simulink model "MVDR_example_hdl_4x4_partial_systolic"  (R2020b)
settings: Solver=FixedStepDiscrete  StartTime=0.0  StopTime=stoptime  RelTol=1e-3
InitFcn:
  | model_init
values from neighbouring files (symbols this model uses):
  movavg_bitshift = nextpow2(sqrt(windowSize))    [model_init.m]
  mvdrPipelineDelay = covMatDelay+movAvgDelay+matrixDivDelay+normResponseDelay    [model_init.m]
  numArrayElements = 4    [model_init.m]
  srcAngles = [20 60]    [model_init.m]
  sv = step(steeringVector,fc,[scanAngle; 0])    [model_init.m]
  Ts = 1/fs    (= 7.8125e-09)    [model_init.m]
  windowSize = 1024    [model_init.m]
libraries: hdlsllib x11, simulink x4, commfilt2 x4, commrfcorlib x3, commsync2 x3, commrflib2 x2, commrandsrc3 x2, phasedtxrxlib x2, commdigbbndcpm2 x1, embsystolicmatrixops x1, embreciprocals x1, commdigbbndpm3 x1
Description:
  | MVDR HDL 4x4 systolic testbench
settings Model: DataTypeOverride=Off  Creator=The MathWorks, Inc.  LastModifiedBy=tmealey
settings DataIOCC: LimitDataPoints=on  SaveFormat=Array  SaveOutput=off  SaveTime=off  ReturnWorkspaceOutputs=off
settings OptimizationCC: BlockReduction=off  ConditionallyExecuteInputs=off  DefaultParameterBehavior=Inlined  LifeSpan=inf
settings DebuggingCC: ReadBeforeWriteMsg=DisableAll  WriteAfterWriteMsg=DisableAll  WriteAfterReadMsg=DisableAll  AlgebraicLoopMsg=error  UnderspecifiedInitializationDetection=Classic  MergeDetectMultiDrivingBlocksExec=none  SolverPrmCheckMsg=warning  SingleTaskRateTransMsg=error  ParameterPrecisionLossMsg=none  AllowSymbolicDim=off  SFUnexpectedBacktrackingDiag=warning  SFNoUnconditionalDefaultTransitionDiag=warning  SFExecutionAtInitializationDiag=none  ArithmeticOperatorsInVariantConditions=warning
settings HardwareCC: ProdBitPerPointer=32  ProdBitPerSizeT=32  ProdBitPerPtrDiffT=32  ProdLargestAtomicFloat=None  ProdIntDivRoundTo=Undefined  ProdEndianess=Unspecified  ProdWordSize=32  ProdHWDeviceType=ASIC/FPGA->ASIC/FPGA  TargetBitPerPointer=64  TargetBitPerSizeT=64  TargetBitPerPtrDiffT=64  TargetLongLongMode=on  TargetIntDivRoundTo=Zero  TargetEndianess=LittleEndian  TargetWordSize=64  TargetHWDeviceType=Custom Processor->MATLAB Host Computer  ProdEqTarget=off
settings ModelReferenceCC: PropagateSignalLabelsOutOfModel=off
settings SFSimCC: SimUseLocalCustomCode=off  CustomCodeUndefinedFunction=UseInterfaceOnly
settings RTWCC: RTWUseLocalCustomCode=off
settings CodeAppCC: StateflowObjectComments=on
settings GRTTargetCC: TargetLangStandard=C89/C90 (ANSI)
settings ConfigComp: CovMetricSettings=dw  CovSaveCumulativeToWorkspaceVar=on  CovSaveSingleToWorkspaceVar=on  CovExternalEMLEnable=off  CovSFcnEnable=off

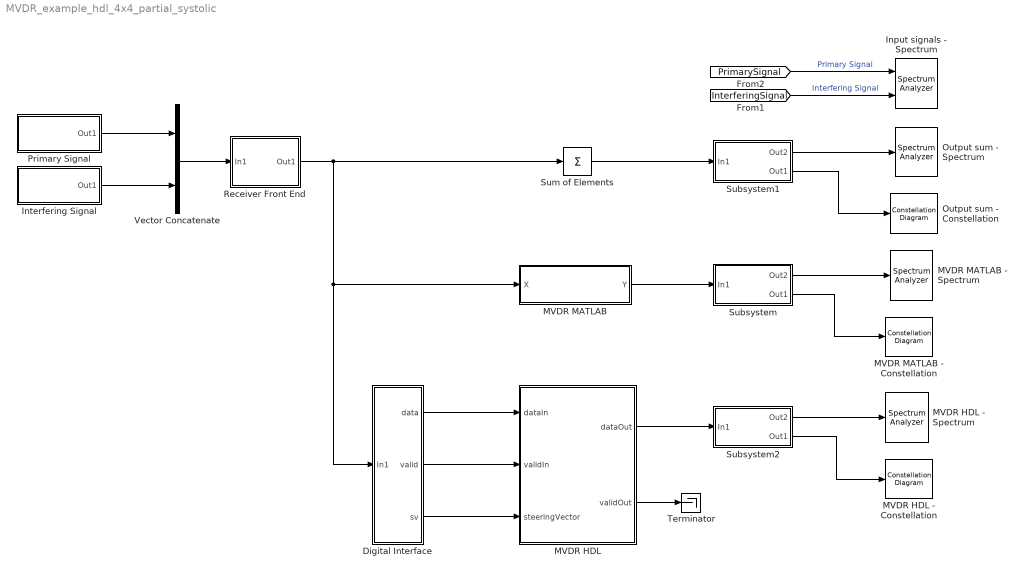
== system MVDR_example_hdl_4x4_partial_systolic ==
  Digital Interface : Subsystem
  Input signals - Spectrum : SpectrumAnalyzer  NumInputPorts=2
  Interfering Signal : Subsystem
      mask Display: disp('Interfering\nSignal')
  MVDR HDL : Subsystem
  MVDR HDL - Constellation : ConstellationDiagram
  MVDR HDL - Spectrum : SpectrumAnalyzer
  MVDR MATLAB : Subsystem
  MVDR MATLAB - Constellation : ConstellationDiagram
  MVDR MATLAB - Spectrum : SpectrumAnalyzer
  Output sum - Constellation : ConstellationDiagram
  Output sum - Spectrum : SpectrumAnalyzer
  Primary Signal : Subsystem
      mask Display: disp('Primary\nSignal')
  Receiver Front End : Subsystem
  Subsystem : Subsystem
  Subsystem1 : Subsystem
  Subsystem2 : Subsystem
  Sum of Elements : Sum  Inputs=+  CollapseMode=Specified dimension  CollapseDim=2
  Terminator : Terminator
  Vector Concatenate : Concatenate  Mode=Multidimensional array  ConcatenateDimension=2
  wires:
  MVDR HDL/2(validOut) -> Terminator/1
  MVDR MATLAB/1(Y) -> Subsystem/1(In1)
  Interfering Signal/1(Out1) -> Vector Concatenate/2
  Primary Signal/1(Out1) -> Vector Concatenate/1
  [InterferingSignal] -> Input signals - Spectrum/2  "Interfering Signal"
  Subsystem/2(Out1) -> MVDR MATLAB - Constellation/1
  Subsystem/1(Out2) -> MVDR MATLAB - Spectrum/1
  Sum of Elements/1 -> Subsystem1/1(In1)
  Subsystem1/1(Out2) -> Output sum - Spectrum/1
  Subsystem1/2(Out1) -> Output sum - Constellation/1
  MVDR HDL/1(dataOut) -> Subsystem2/1(In1)
  Subsystem2/1(Out2) -> MVDR HDL - Spectrum/1
  Subsystem2/2(Out1) -> MVDR HDL - Constellation/1
  [PrimarySignal] -> Input signals - Spectrum/1  "Primary Signal"
  Digital Interface/1(data) -> MVDR HDL/1(dataIn)
  Digital Interface/2(valid) -> MVDR HDL/2(validIn)
  Digital Interface/3(sv) -> MVDR HDL/3(steeringVector)
  Receiver Front End/1(Out1) -> MVDR MATLAB/1(X), Digital Interface/1(In1), Sum of Elements/1
  Vector Concatenate/1 -> Receiver Front End/1(In1)

== system MVDR_example_hdl_4x4_partial_systolic/Digital Interface ==
  In1 : Inport
  Constant1 : Constant  Value=true  SampleTime=-1
  Constant2 : Constant  Value=sv  SampleTime=-1
  Data Type Conversion : DataTypeConversion  OutDataTypeStr=sv_dt
  Input DTC : Subsystem
  Unbuffer : Unbuffer
  data : Outport
  valid : Outport  Port=2
  sv : Outport  Port=3
  wires:
  Unbuffer/1 -> Input DTC/1(In1)
  Constant2/1 -> Data Type Conversion/1
  In1/1 -> Unbuffer/1
  Data Type Conversion/1 -> sv/1
  Constant1/1 -> valid/1
  Input DTC/1(Out1) -> data/1

== system MVDR_example_hdl_4x4_partial_systolic/Interfering Signal ==
  GMSK Modulator Baseband : commdigbbndcpm2/GMSK Modulator Baseband  inputType=Bit  BT=.3  pulseLength=4  preHistory=1  phaseOffset=0  samplesPerSymbol=8  RateOptions=Enforce single-rate processing  outDataType=double
      settings: SourceProductBaseCode=CM
  Gain : Gain  Gain=1/40
  Memoryless Nonlinearity2 : commrflib2/Memoryless Nonlinearity  model_select=Cubic polynomial  linGaindB=39  GindB=0  iip3=43  am2pm=.8  LPwrLimAMPM=-2.5  UPwrLimAMPM=17.5  amam=[2.1587 1.1517]  ampm=[4.0033 9.1040]  x=[8.1081 1.5413 6.5202 -0.0718]  y=[4.6645 2.0965 10.88 -0.003]  p=0.5  GoutdB=0  vsat=1
      settings: SourceProductBaseCode=CM
  Random Integer Generator1 : commrandsrc3/Random Integer Generator  SetSize=2  SeedSource=Auto  Seed=0  SampleTime=4*Ts  SamplesPerFrame=100  OutputDataType=boolean  SimulateUsing=Interpreted execution
  Out1 : Outport  VectorParamsAs1DForOutWhenUnconnected=off
  tag scope: InterferingSignal=global
  wires:
  Memoryless Nonlinearity2/1 -> Gain/1
  GMSK Modulator Baseband/1 -> Memoryless Nonlinearity2/1
  Random Integer Generator1/1 -> GMSK Modulator Baseband/1
  Gain/1 -> Out1/1, [InterferingSignal]

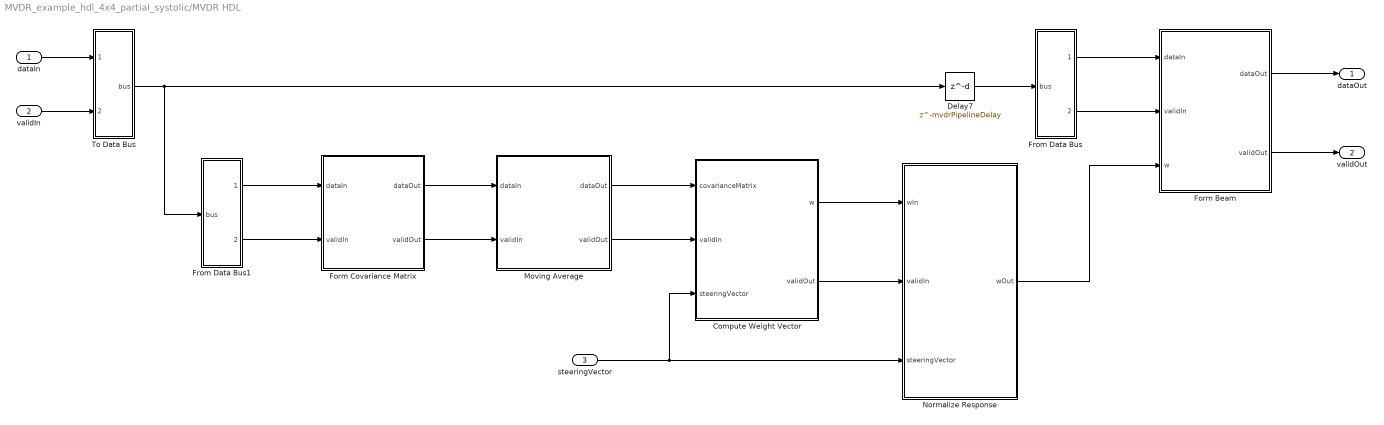
== system MVDR_example_hdl_4x4_partial_systolic/MVDR HDL ==
  dataIn : Inport
  validIn : Inport  Port=2
  steeringVector : Inport  Port=3
  Compute Weight Vector : Subsystem
  Delay7 : Delay  DelayLength=mvdrPipelineDelay
  Form Beam : Subsystem
  Form Covariance Matrix : Subsystem
  From Data Bus : Subsystem
  From Data Bus1 : Subsystem
  Moving Average : Subsystem
  Normalize Response : Subsystem
  To Data Bus : Subsystem
  dataOut : Outport
  validOut : Outport  Port=2
  wires:
  validIn/1 -> To Data Bus/2(valid)
  Normalize Response/1(wOut) -> Form Beam/3(w)
  Form Beam/1(dataOut) -> dataOut/1
  Form Covariance Matrix/2(validOut) -> Moving Average/2(validIn)
  Form Beam/2(validOut) -> validOut/1
  Compute Weight Vector/1(w) -> Normalize Response/1(wIn)
  steeringVector/1 -> Compute Weight Vector/3(steeringVector), Normalize Response/3(steeringVector)
  dataIn/1 -> To Data Bus/1(data)
  Form Covariance Matrix/1(dataOut) -> Moving Average/1(dataIn)
  Moving Average/1(dataOut) -> Compute Weight Vector/1(covarianceMatrix)
  To Data Bus/1(bus) -> Delay7/1, From Data Bus1/1(bus)
  Moving Average/2(validOut) -> Compute Weight Vector/2(validIn)
  Compute Weight Vector/2(validOut) -> Normalize Response/2(validIn)
  Delay7/1 -> From Data Bus/1(bus)
  From Data Bus/1(data) -> Form Beam/1(dataIn)
  From Data Bus/2(valid) -> Form Beam/2(validIn)
  From Data Bus1/1(data) -> Form Covariance Matrix/1(dataIn)
  From Data Bus1/2(valid) -> Form Covariance Matrix/2(validIn)

== system MVDR_example_hdl_4x4_partial_systolic/MVDR MATLAB ==
  X : Inport
  MATLAB Function : MATLAB Function  TreatAsAtomicUnit=on
  Y : Outport
  wires:
  MATLAB Function/1(Y) -> Y/1
  X/1 -> MATLAB Function/1(X)

== system MVDR_example_hdl_4x4_partial_systolic/Primary Signal ==
  Gain : Gain  Gain=1/40
  Memoryless Nonlinearity : commrflib2/Memoryless Nonlinearity  model_select=Cubic polynomial  linGaindB=28  GindB=0  iip3=43  am2pm=.8  LPwrLimAMPM=-2.5  UPwrLimAMPM=17.5  amam=[2.1587 1.1517]  ampm=[4.0033 9.1040]  x=[8.1081 1.5413 6.5202 -0.0718]  y=[4.6645 2.0965 10.88 -0.003]  p=0.5  GoutdB=0  vsat=1
      settings: SourceProductBaseCode=CM
  QPSK Modulator Baseband : commdigbbndpm3/QPSK Modulator Baseband  InType=Integer  Enc=Gray  Ph=pi/4  outDtype=double  outWordLen=16  outUDDataType=sfix(16)  outFracLenMode=Best precision  outFracLen=15  outDataTypeStr=double  outLastDataTypeStr=double
  Raised Cosine Transmit Filter : commfilt2/Raised Cosine Transmit Filter  filtType=Square root  R=.3  filtSpan=10  N=2  filterGain=1  InputProcessing=Columns as channels (frame based)  RateOptions=Enforce single-rate processing  framing=Mute  checkCoeff=off  variableName=rcTxFilt  checkGain=Normalized  sampMode=Mute  saveAsFlag=0  currentFiltSpan=10  D=(10)/2  launchFVT=on  roundingMode=Floor  overflowMode=off  coeffDataTypeStr=Inherit: Same word length as input  coeffMin=[]  coeffMax=[]  coeffLastDataTypeStr=Inherit: Same word length as input  outputDataTypeStr=Inherit: Same as accumulator  outputMin=[]  outputMax=[]  outputLastDataTypeStr=Inherit: Same as accumulator
  Random Integer Generator : commrandsrc3/Random Integer Generator  SetSize=4  SeedSource=Auto  Seed=0  SampleTime=Ts  SamplesPerFrame=400  OutputDataType=double  SimulateUsing=Interpreted execution
  Out1 : Outport  VectorParamsAs1DForOutWhenUnconnected=off
  tag scope: PrimarySignal=global
  wires:
  QPSK Modulator Baseband/1 -> Raised Cosine Transmit Filter/1
  Random Integer Generator/1 -> QPSK Modulator Baseband/1
  Memoryless Nonlinearity/1 -> Gain/1
  Raised Cosine Transmit Filter/1 -> Memoryless Nonlinearity/1
  Gain/1 -> Out1/1, [PrimarySignal]

== system MVDR_example_hdl_4x4_partial_systolic/Receiver Front End ==
  In1 : Inport
  Constant : Constant  Value=srcAngles  SampleTime=-1
  Narrowband Receive Array : phasedtxrxlib/Narrowband Receive Array  PropagationSpeed=propSpeed  OperatingFrequency=fc  Wavefront=Plane  SensorGainMeasure=dB  Polarization=None  WeightsInputPort=off  SimulateUsing=Interpreted execution  Sensor=sensorArray
      settings: SourceProductBaseCode=AR
  Receiver Preamp : phasedtxrxlib/Receiver Preamp  Gain=-10  LossFactor=0  NoiseMethod=Noise power  NoiseFigure=0  ReferenceTemperature=290  SampleRateFromInputCheckbox=on  SampleRate=1e6  NoisePower=.001  EnableInputPort=off  PhaseNoiseInputPort=off  SeedSource=Auto  Seed=0  SimulateUsing=Interpreted execution
      settings: SourceProductBaseCode=AR
  Reshape : Reshape  OutputDimensionality=Row vector (2-D)
  Out1 : Outport
  wires:
  In1/1 -> Narrowband Receive Array/1
  Narrowband Receive Array/1 -> Receiver Preamp/1
  Constant/1 -> Reshape/1
  Reshape/1 -> Narrowband Receive Array/2
  Receiver Preamp/1 -> Out1/1

== system MVDR_example_hdl_4x4_partial_systolic/Subsystem ==
  In1 : Inport
  AGC : commrfcorlib/AGC  LegacyMode=off  DetectorMethod=Rectifier  LoopMethod=Linear  UpdatePeriod=100  StepSize=0.1  AdaptationStepSize=0.01  DesiredOutputPower=1  AveragingLength=200  MaximumGain=30  MaxPowerGain=60  GainOutputPort=off  InputPowerOutputPort=off  SimulateUsing=Interpreted execution
  Carrier Synchronizer : commsync2/Carrier Synchronizer  Modulation=QPSK  ModulationPhaseOffset=Auto  CustomPhaseOffset=0  SamplesPerSymbol=1  DampingFactor=0.707  NormalizedLoopBandwidth=0.01  EstimatedPhaseErrorOutputPort=off  SimulateUsing=Interpreted execution
  Raised Cosine Receive Filter : commfilt2/Raised Cosine Receive Filter  filtType=Square root  R=.3  filtSpan=10  N=2  downFactor=2  downOffset=0  filterGain=1  InputProcessing=Columns as channels (frame based)  RateOptions=Enforce single-rate processing  framing=Mute  checkCoeff=off  variableName=rcRxFilt  currentFiltSpan=10  D=5  inputOffset=0  sampMode=Mute  saveAsFlag=0  rateMode=Downsampling  checkGain=Normalized  launchFVT=on  roundingMode=Floor  overflowMode=off  coeffDataTypeStr=Inherit: Same word length as input  coeffMin=[]  coeffMax=[]  coeffLastDataTypeStr=Inherit: Same word length as input  accumDataTypeStr=Inherit: Same as product output  accumLastDataTypeStr=Inherit: Same as product output  outputDataTypeStr=Inherit: Same as accumulator  outputMin=[]  outputMax=[]  outputLastDataTypeStr=Inherit: Same as accumulator
  Out2 : Outport
  Out1 : Outport  Port=2
  wires:
  In1/1 -> Out2/1, Raised Cosine Receive Filter/1
  Raised Cosine Receive Filter/1 -> Carrier Synchronizer/1
  AGC/1 -> Out1/1
  Carrier Synchronizer/1 -> AGC/1

== system MVDR_example_hdl_4x4_partial_systolic/Subsystem1 ==
  In1 : Inport
  AGC : commrfcorlib/AGC  LegacyMode=off  DetectorMethod=Rectifier  LoopMethod=Linear  UpdatePeriod=100  StepSize=0.1  AdaptationStepSize=0.01  DesiredOutputPower=1  AveragingLength=200  MaximumGain=30  MaxPowerGain=60  GainOutputPort=off  InputPowerOutputPort=off  SimulateUsing=Interpreted execution
  Carrier Synchronizer : commsync2/Carrier Synchronizer  Modulation=QPSK  ModulationPhaseOffset=Auto  CustomPhaseOffset=0  SamplesPerSymbol=1  DampingFactor=0.707  NormalizedLoopBandwidth=0.01  EstimatedPhaseErrorOutputPort=off  SimulateUsing=Interpreted execution
  Raised Cosine Receive Filter : commfilt2/Raised Cosine Receive Filter  filtType=Square root  R=.3  filtSpan=10  N=2  downFactor=2  downOffset=0  filterGain=1  InputProcessing=Columns as channels (frame based)  RateOptions=Enforce single-rate processing  framing=Mute  checkCoeff=off  variableName=rcRxFilt  currentFiltSpan=10  D=5  inputOffset=0  sampMode=Mute  saveAsFlag=0  rateMode=Downsampling  checkGain=Normalized  launchFVT=on  roundingMode=Floor  overflowMode=off  coeffDataTypeStr=Inherit: Same word length as input  coeffMin=[]  coeffMax=[]  coeffLastDataTypeStr=Inherit: Same word length as input  accumDataTypeStr=Inherit: Same as product output  accumLastDataTypeStr=Inherit: Same as product output  outputDataTypeStr=Inherit: Same as accumulator  outputMin=[]  outputMax=[]  outputLastDataTypeStr=Inherit: Same as accumulator
  Out2 : Outport
  Out1 : Outport  Port=2
  wires:
  Carrier Synchronizer/1 -> AGC/1
  AGC/1 -> Out1/1
  Raised Cosine Receive Filter/1 -> Carrier Synchronizer/1
  In1/1 -> Raised Cosine Receive Filter/1, Out2/1

== system MVDR_example_hdl_4x4_partial_systolic/Subsystem2 ==
  In1 : Inport
  AGC : commrfcorlib/AGC  LegacyMode=off  DetectorMethod=Rectifier  LoopMethod=Linear  UpdatePeriod=100  StepSize=0.1  AdaptationStepSize=0.01  DesiredOutputPower=1  AveragingLength=200  MaximumGain=30  MaxPowerGain=60  GainOutputPort=off  InputPowerOutputPort=off  SimulateUsing=Interpreted execution
  Buffer : Buffer  N=800  OutputFrames=off
  Carrier Synchronizer : commsync2/Carrier Synchronizer  Modulation=QPSK  ModulationPhaseOffset=Auto  CustomPhaseOffset=0  SamplesPerSymbol=1  DampingFactor=0.707  NormalizedLoopBandwidth=0.01  EstimatedPhaseErrorOutputPort=off  SimulateUsing=Interpreted execution
  Data Type Conversion : DataTypeConversion  OutDataTypeStr=double
  Raised Cosine Receive Filter : commfilt2/Raised Cosine Receive Filter  filtType=Square root  R=.3  filtSpan=10  N=2  downFactor=2  downOffset=0  filterGain=1  InputProcessing=Columns as channels (frame based)  RateOptions=Enforce single-rate processing  framing=Mute  checkCoeff=off  variableName=rcRxFilt  currentFiltSpan=10  D=5  inputOffset=0  sampMode=Mute  saveAsFlag=0  rateMode=Downsampling  checkGain=Normalized  launchFVT=on  roundingMode=Floor  overflowMode=off  coeffDataTypeStr=Inherit: Same word length as input  coeffMin=[]  coeffMax=[]  coeffLastDataTypeStr=Inherit: Same word length as input  accumDataTypeStr=Inherit: Same as product output  accumLastDataTypeStr=Inherit: Same as product output  outputDataTypeStr=Inherit: Same as accumulator  outputMin=[]  outputMax=[]  outputLastDataTypeStr=Inherit: Same as accumulator
  Out2 : Outport
  Out1 : Outport  Port=2
  wires:
  Carrier Synchronizer/1 -> AGC/1
  AGC/1 -> Out1/1
  Raised Cosine Receive Filter/1 -> Carrier Synchronizer/1
  In1/1 -> Buffer/1
  Buffer/1 -> Data Type Conversion/1
  Data Type Conversion/1 -> Raised Cosine Receive Filter/1, Out2/1

== system MVDR_example_hdl_4x4_partial_systolic/Digital Interface/Input DTC ==
  In1 : Inport
  Data Type Conversion : DataTypeConversion  OutDataTypeStr=input_dt
  Data Type Conversion1 : DataTypeConversion  OutDataTypeStr=adc_dt
  Out1 : Outport
  wires:
  Data Type Conversion/1 -> Out1/1
  In1/1 -> Data Type Conversion1/1
  Data Type Conversion1/1 -> Data Type Conversion/1

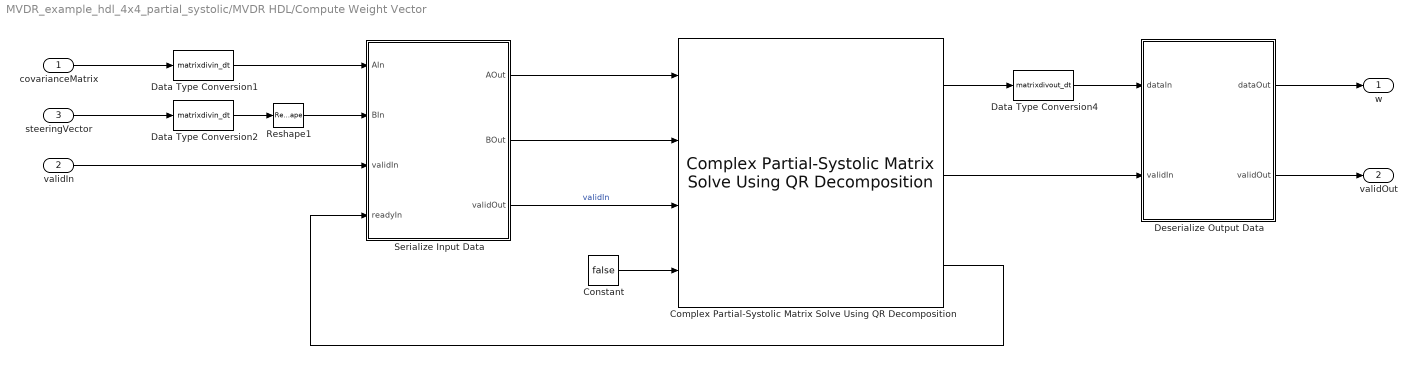
== system MVDR_example_hdl_4x4_partial_systolic/MVDR HDL/Compute Weight Vector ==
  covarianceMatrix : Inport
  validIn : Inport  Port=2
  steeringVector : Inport  Port=3
  Complex Partial-Systolic Matrix Solve Using QR Decomposition : embsystolicmatrixops/Complex Partial-Systolic Matrix Solve Using QR Decomposition  m=4  n=4  p=1  regularizationParameter=0  OutputType=fixdt(1,32,15)
      settings: SourceProductBaseCode=SL
  Constant : Constant  Value=false  SampleTime=-1
  Data Type Conversion1 : DataTypeConversion  OutDataTypeStr=matrixdivin_dt
  Data Type Conversion2 : DataTypeConversion  OutDataTypeStr=matrixdivin_dt
  Data Type Conversion4 : DataTypeConversion  OutDataTypeStr=matrixdivout_dt
  Deserialize Output Data : Subsystem
  Reshape1 : Reshape  OutputDimensionality=Column vector (2-D)  OutputDimensions=[4,4]
  Serialize Input Data : Subsystem
  w : Outport
  validOut : Outport  Port=2
  wires:
  covarianceMatrix/1 -> Data Type Conversion1/1
  steeringVector/1 -> Data Type Conversion2/1
  Data Type Conversion2/1 -> Reshape1/1
  validIn/1 -> Serialize Input Data/3(validIn)
  Constant/1 -> Complex Partial-Systolic Matrix Solve Using QR Decomposition/4
  Serialize Input Data/3(validOut) -> Complex Partial-Systolic Matrix Solve Using QR Decomposition/3  "validIn"
  Complex Partial-Systolic Matrix Solve Using QR Decomposition/3 -> Serialize Input Data/4(readyIn)
  Serialize Input Data/1(AOut) -> Complex Partial-Systolic Matrix Solve Using QR Decomposition/1
  Reshape1/1 -> Serialize Input Data/2(BIn)
  Complex Partial-Systolic Matrix Solve Using QR Decomposition/1 -> Data Type Conversion4/1
  Data Type Conversion4/1 -> Deserialize Output Data/1(dataIn)
  Complex Partial-Systolic Matrix Solve Using QR Decomposition/2 -> Deserialize Output Data/2(validIn)
  Deserialize Output Data/1(dataOut) -> w/1
  Deserialize Output Data/2(validOut) -> validOut/1
  Serialize Input Data/2(BOut) -> Complex Partial-Systolic Matrix Solve Using QR Decomposition/2
  Data Type Conversion1/1 -> Serialize Input Data/1(AIn)

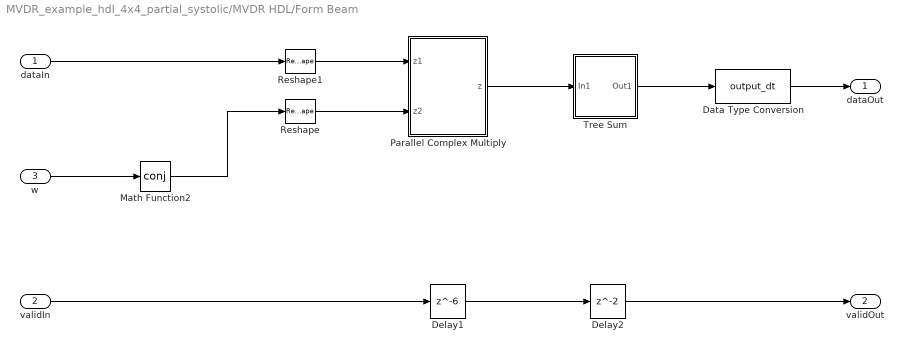
== system MVDR_example_hdl_4x4_partial_systolic/MVDR HDL/Form Beam ==
  dataIn : Inport
  validIn : Inport  Port=2
  w : Inport  Port=3
  Data Type Conversion : DataTypeConversion  OutDataTypeStr=output_dt
  Delay1 : Delay  DelayLength=6
  Delay2 : Delay
  Math Function2 : Math  Operator=conj  SaturateOnIntegerOverflow=on
  Parallel Complex Multiply : Subsystem  TreatAsAtomicUnit=on
  Reshape : Reshape
  Reshape1 : Reshape
  Tree Sum : Subsystem
  dataOut : Outport
  validOut : Outport  Port=2
  wires:
  dataIn/1 -> Reshape1/1
  Parallel Complex Multiply/1(z) -> Tree Sum/1(In1)
  Tree Sum/1(Out1) -> Data Type Conversion/1
  Math Function2/1 -> Reshape/1
  w/1 -> Math Function2/1
  validIn/1 -> Delay1/1
  Reshape/1 -> Parallel Complex Multiply/2(z2)
  Reshape1/1 -> Parallel Complex Multiply/1(z1)
  Data Type Conversion/1 -> dataOut/1
  Delay2/1 -> validOut/1
  Delay1/1 -> Delay2/1

== system MVDR_example_hdl_4x4_partial_systolic/MVDR HDL/Form Covariance Matrix ==
  dataIn : Inport
  validIn : Inport  Port=2
  Conj : Math  Operator=conj
  Data Type Conversion : DataTypeConversion  OutDataTypeStr=covmat_dt
  Data Type Conversion1 : DataTypeConversion  OutDataTypeStr=adc_dt
  Delay : Delay  DelayLength=6
  Matrix Multiply Partitioned : Subsystem  TreatAsAtomicUnit=on
  Reshape : Reshape
  dataOut : Outport
  validOut : Outport  Port=2
  wires:
  validIn/1 -> Delay/1
  dataIn/1 -> Data Type Conversion1/1
  Reshape/1 -> Conj/1, Matrix Multiply Partitioned/1(x)  "x"
  Matrix Multiply Partitioned/1(C) -> Data Type Conversion/1  "x * x'"
  Delay/1 -> validOut/1
  Conj/1 -> Matrix Multiply Partitioned/2(x_conj)
  Data Type Conversion1/1 -> Reshape/1
  Data Type Conversion/1 -> dataOut/1

== system MVDR_example_hdl_4x4_partial_systolic/MVDR HDL/From Data Bus ==
  bus : Inport
  Bus Selector : BusSelector  OutputSignals=data,valid
  data : Outport
  valid : Outport  Port=2
  wires:
  Bus Selector/2 -> valid/1  "<valid>"
  Bus Selector/1 -> data/1  "<data>"
  bus/1 -> Bus Selector/1

== system MVDR_example_hdl_4x4_partial_systolic/MVDR HDL/From Data Bus1 ==
  bus : Inport
  Bus Selector : BusSelector  OutputSignals=data,valid
  data : Outport
  valid : Outport  Port=2
  wires:
  bus/1 -> Bus Selector/1
  Bus Selector/1 -> data/1  "<data>"
  Bus Selector/2 -> valid/1  "<valid>"

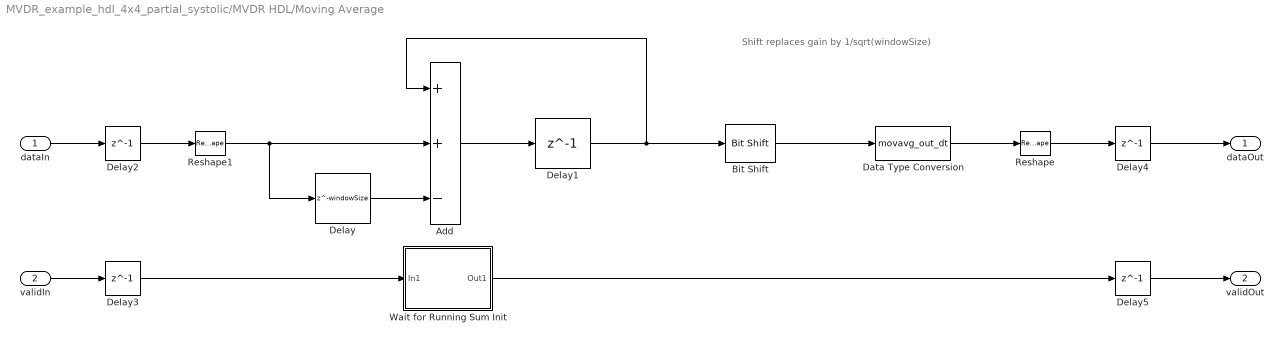
== system MVDR_example_hdl_4x4_partial_systolic/MVDR HDL/Moving Average ==
  note: Shift replaces gain by 1/sqrt(windowSize)
  dataIn : Inport
  validIn : Inport  Port=2
  Add : Sum  Inputs=++-  AccumDataTypeStr=movavg_accum_dt  OutDataTypeStr=Inherit: Same as accumulator
  Bit Shift : hdlsllib/Logic and Bit Operations/Bit Shift  mode=Shift Right Arithmetic  N=movavg_bitshift
  Data Type Conversion : DataTypeConversion  OutDataTypeStr=movavg_out_dt
  Delay : Delay  DelayLength=windowSize
  Delay{1..5} (5 alike) : Delay  DelayLength=1
  Reshape : Reshape  OutputDimensionality=Customize  OutputDimensions=[4,4]
  Reshape1 : Reshape  OutputDimensions=[4,4]
  Wait for Running Sum Init : Subsystem
  dataOut : Outport
  validOut : Outport  Port=2
  wires:
  Bit Shift/1 -> Data Type Conversion/1
  Delay1/1 -> Bit Shift/1, Add/1
  Delay/1 -> Add/3
  Add/1 -> Delay1/1
  dataIn/1 -> Delay2/1
  validIn/1 -> Delay3/1
  Delay2/1 -> Reshape1/1
  Delay4/1 -> dataOut/1
  Delay5/1 -> validOut/1
  Delay3/1 -> Wait for Running Sum Init/1(In1)
  Wait for Running Sum Init/1(Out1) -> Delay5/1
  Data Type Conversion/1 -> Reshape/1
  Reshape/1 -> Delay4/1
  Reshape1/1 -> Delay/1, Add/2

== system MVDR_example_hdl_4x4_partial_systolic/MVDR HDL/Normalize Response ==
  note: This subsystem scales the weight vector to ensure unit gain in the target direction.
  wIn : Inport
  validIn : Inport  Port=2
  steeringVector : Inport  Port=3
  MVDR Weight Update : Subsystem
  Unit Delay Enabled Synchronous : hdlsllib/Discrete/Unit Delay Enabled Synchronous  InitialCondition=0.0  SampleTime=-1
      settings: SourceProductBaseCode=SL
  wOut : Outport
  wires:
  steeringVector/1 -> MVDR Weight Update/1(Steering Vector)
  wIn/1 -> MVDR Weight Update/2(x)
  MVDR Weight Update/1(w) -> Unit Delay Enabled Synchronous/1
  MVDR Weight Update/2(validOut) -> Unit Delay Enabled Synchronous/2
  Unit Delay Enabled Synchronous/1 -> wOut/1
  validIn/1 -> MVDR Weight Update/3(validIn)

== system MVDR_example_hdl_4x4_partial_systolic/MVDR HDL/To Data Bus ==
  data : Inport
  valid : Inport  Port=2
  Bus Creator : BusCreator  Inputs=2
  bus : Outport
  wires:
  data/1 -> Bus Creator/1  "data"
  Bus Creator/1 -> bus/1
  valid/1 -> Bus Creator/2  "valid"

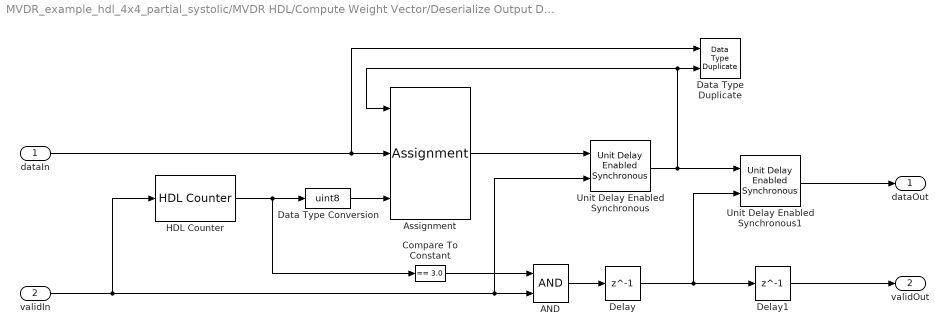
== system MVDR_example_hdl_4x4_partial_systolic/MVDR HDL/Compute Weight Vector/Deserialize Output Data ==
  dataIn : Inport
  validIn : Inport  Port=2
  AND : Logic  IconShape=distinctive  AllPortsSameDT=off  OutDataTypeStr=boolean
  Assignment : Assignment  IndexMode=Zero-based  DiagnosticForDimensions=Warning  IndexOptions=Index vector (port)  Indices=1  OutputSizes=4
  Compare To Constant : simulink/Logic and Bit Operations/Compare To Constant  relop===  const=3.0  OutDataTypeStr=boolean
  Data Type Duplicate : DataTypeDuplicate
  Data Type Conversion : DataTypeConversion  OutDataTypeStr=uint8
  Delay : Delay  DelayLength=1
  Delay1 : Delay  DelayLength=1
  HDL Counter : hdlsllib/Sources/HDL Counter  CountType=Free running  CountInit=0  CountStep=1  CountMax=25  CountFromType=Initial value  CountFrom=0  CountResetPort=off  CountLoadPort=off  CountEnbPort=on  CountDirPort=off  CountDataType=Unsigned  CountWordLen=2  CountFracLen=0  CountSampTime=1
  Unit Delay Enabled Synchronous : hdlsllib/Discrete/Unit Delay Enabled Synchronous  InitialCondition=complex(zeros(4,1))  SampleTime=-1
      settings: SourceProductBaseCode=SL
  Unit Delay Enabled Synchronous1 : hdlsllib/Discrete/Unit Delay Enabled Synchronous  InitialCondition=0  SampleTime=-1
      settings: SourceProductBaseCode=SL
  dataOut : Outport
  validOut : Outport  Port=2
  wires:
  AND/1 -> Delay/1
  HDL Counter/1 -> Compare To Constant/1, Data Type Conversion/1
  dataIn/1 -> Data Type Duplicate/1, Assignment/2
  Compare To Constant/1 -> AND/1
  Delay/1 -> Delay1/1, Unit Delay Enabled Synchronous1/2
  Data Type Conversion/1 -> Assignment/3
  validIn/1 -> HDL Counter/1, Unit Delay Enabled Synchronous/2, AND/2
  Assignment/1 -> Unit Delay Enabled Synchronous/1
  Unit Delay Enabled Synchronous/1 -> Assignment/1, Data Type Duplicate/2, Unit Delay Enabled Synchronous1/1
  Delay1/1 -> validOut/1
  Unit Delay Enabled Synchronous1/1 -> dataOut/1

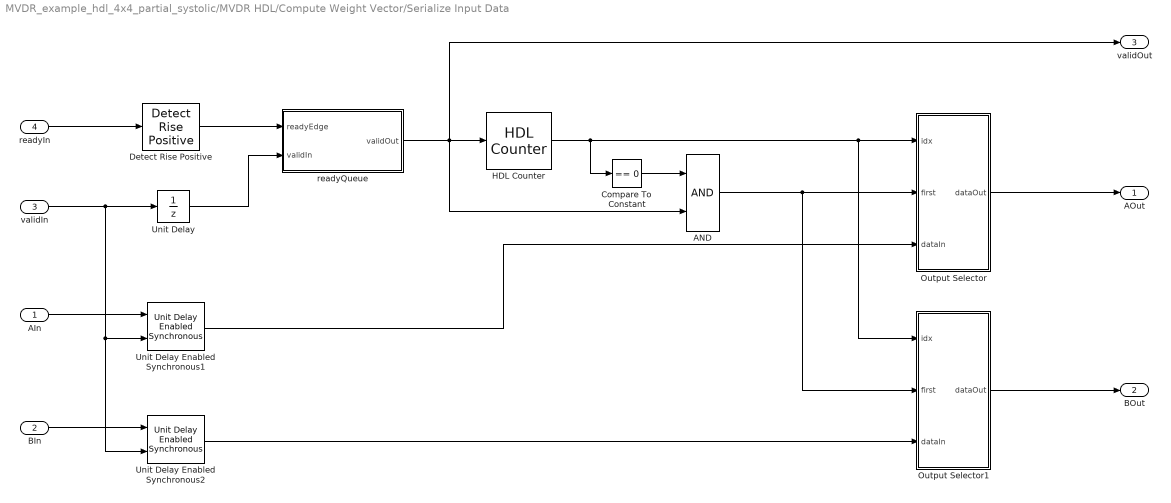
== system MVDR_example_hdl_4x4_partial_systolic/MVDR HDL/Compute Weight Vector/Serialize Input Data ==
  AIn : Inport
  BIn : Inport  Port=2
  validIn : Inport  Port=3
  readyIn : Inport  Port=4
  AND : Logic  IconShape=distinctive  AllPortsSameDT=off  OutDataTypeStr=boolean
  Compare To Constant : simulink/Logic and Bit Operations/Compare To Constant  relop===  const=0  OutDataTypeStr=boolean
  Detect Rise Positive : simulink/Logic and Bit Operations/Detect Rise Positive  vinit=0  OutDataTypeStr=boolean
  HDL Counter : hdlsllib/Sources/HDL Counter  CountType=Free running  CountInit=0  CountStep=1  CountMax=25  CountFromType=Initial value  CountFrom=0  CountResetPort=off  CountLoadPort=off  CountEnbPort=on  CountDirPort=off  CountDataType=Unsigned  CountWordLen=2  CountFracLen=0  CountSampTime=1
  Output Selector : Subsystem
  Output Selector1 : Subsystem
  Unit Delay : UnitDelay  SampleTime=-1  HasFrameUpgradeWarning=on
  Unit Delay Enabled Synchronous1 : hdlsllib/Discrete/Unit Delay Enabled Synchronous  InitialCondition=0.0  SampleTime=-1
      settings: SourceProductBaseCode=SL
  Unit Delay Enabled Synchronous2 : hdlsllib/Discrete/Unit Delay Enabled Synchronous  InitialCondition=0.0  SampleTime=-1
      settings: SourceProductBaseCode=SL
  readyQueue : MATLAB Function  TreatAsAtomicUnit=on
  AOut : Outport
  BOut : Outport  Port=2
  validOut : Outport  Port=3
  wires:
  readyIn/1 -> Detect Rise Positive/1
  HDL Counter/1 -> Compare To Constant/1, Output Selector1/1(idx), Output Selector/1(idx)
  Compare To Constant/1 -> AND/1
  readyQueue/1(validOut) -> HDL Counter/1, AND/2, validOut/1
  Detect Rise Positive/1 -> readyQueue/1(readyEdge)
  AIn/1 -> Unit Delay Enabled Synchronous1/1
  validIn/1 -> Unit Delay Enabled Synchronous2/2, Unit Delay Enabled Synchronous1/2, Unit Delay/1
  Unit Delay/1 -> readyQueue/2(validIn)
  BIn/1 -> Unit Delay Enabled Synchronous2/1
  AND/1 -> Output Selector1/2(first), Output Selector/2(first)
  Unit Delay Enabled Synchronous1/1 -> Output Selector/3(dataIn)
  Output Selector/1(dataOut) -> AOut/1
  Unit Delay Enabled Synchronous2/1 -> Output Selector1/3(dataIn)
  Output Selector1/1(dataOut) -> BOut/1

== system MVDR_example_hdl_4x4_partial_systolic/MVDR HDL/Form Beam/Parallel Complex Multiply ==
  z1 : Inport  Partition=on  PartitionDimension=1  PartitionWidth=1  PartitionOffset=0
  z2 : Inport  Port=2  Partition=on  PartitionDimension=1  PartitionWidth=1  PartitionOffset=0
  For Each : ForEach  DisableCoverage=on
  HDL Complex Multiply : Subsystem  mask(HDL Complex Multiplier (3 Multiply, 5 Add)){D1=2, D2=1, D3=1, D4=1, D5=1}
      mask help:
      | Xilinx devices:
      | - Set D1 = 1 or 2 to trade off speed & FF resources
      | - Set D2-D5 = 1 to fully leverage DSP48 pipelines
      | - Use sync reset
      |
      | Intel FPGAs:
      | - Set D1 = 1 or 2 depending on device family
      | - Set D5 = 1; D2, D3, D4 = 0
      | - Use async reset
      mask init:
      | delay = D1+D2+D3+D4+D5;
      mask Display:
      | fprintf('Delay=%d',delay);
      | port_label('input',1,'z1');
      | port_label('input',2,'z2');
  z : Outport  ConcatenationDimension=1
  wires:
  z1/1 -> HDL Complex Multiply/1(In1)
  z2/1 -> HDL Complex Multiply/2(In2)
  HDL Complex Multiply/1(Out1) -> z/1

== system MVDR_example_hdl_4x4_partial_systolic/MVDR HDL/Form Beam/Tree Sum ==
  In1 : Inport
  Delay3 : Delay  DelayLength=ceil(log2(numArrayElements))
  Tree Sum of Elements : Sum  Inputs=+  OutDataTypeStr=Inherit: Same as first input  LockScale=on
  Out1 : Outport
  wires:
  Delay3/1 -> Out1/1
  In1/1 -> Tree Sum of Elements/1
  Tree Sum of Elements/1 -> Delay3/1

== system MVDR_example_hdl_4x4_partial_systolic/MVDR HDL/Form Covariance Matrix/Matrix Multiply Partitioned ==
  x : Inport
  x_conj : Inport  Port=2
  Partition x_conj : Subsystem
  Reshape : Reshape  OutputDimensionality=Customize  OutputDimensions=[4,4]
  C : Outport
  wires:
  x/1 -> Partition x_conj/1(x)
  x_conj/1 -> Partition x_conj/2(x_conj)
  Partition x_conj/1(C) -> Reshape/1
  Reshape/1 -> C/1

== system MVDR_example_hdl_4x4_partial_systolic/MVDR HDL/Moving Average/Wait for Running Sum Init ==
  In1 : Inport
  Compare To Constant : simulink/Logic and Bit Operations/Compare To Constant  relop=<  const=windowSize  OutDataTypeStr=boolean
  HDL Counter : hdlsllib/Sources/HDL Counter  CountType=Free running  CountInit=0  CountStep=1  CountMax=25  CountFromType=Initial value  CountFrom=0  CountResetPort=off  CountLoadPort=off  CountEnbPort=on  CountDirPort=off  CountDataType=Unsigned  CountWordLen=nextpow2(windowSize)+1  CountFracLen=0  CountSampTime=1
  Logical Operator : Logic  IconShape=distinctive  AllPortsSameDT=off  OutDataTypeStr=boolean
  Logical Operator1 : Logic  IconShape=distinctive  AllPortsSameDT=off  OutDataTypeStr=boolean
  Logical Operator2 : Logic  Operator=NOT  IconShape=distinctive  AllPortsSameDT=off  OutDataTypeStr=boolean
  Out1 : Outport
  wires:
  Logical Operator2/1 -> Logical Operator/2
  Logical Operator1/1 -> HDL Counter/1
  Compare To Constant/1 -> Logical Operator1/2, Logical Operator2/1
  Logical Operator/1 -> Out1/1
  HDL Counter/1 -> Compare To Constant/1
  In1/1 -> Logical Operator1/1, Logical Operator/1

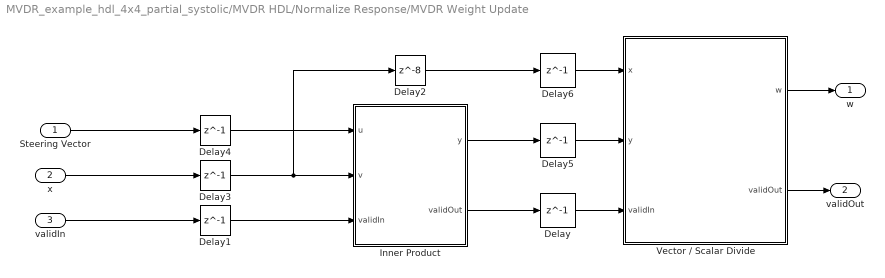
== system MVDR_example_hdl_4x4_partial_systolic/MVDR HDL/Normalize Response/MVDR Weight Update ==
  Steering Vector : Inport
  x : Inport  Port=2
  validIn : Inport  Port=3
  Delay{,1,3..6} (6 alike) : Delay  DelayLength=1
  Delay2 : Delay  DelayLength=8
  Inner Product : Subsystem
  Vector / Scalar Divide : Subsystem
  w : Outport
  validOut : Outport  Port=2
  wires:
  x/1 -> Delay3/1
  Vector / Scalar Divide/1(w) -> w/1
  Delay4/1 -> Inner Product/1(u)
  Inner Product/1(y) -> Delay5/1
  Delay6/1 -> Vector / Scalar Divide/1(x)
  Delay/1 -> Vector / Scalar Divide/3(validIn)
  Steering Vector/1 -> Delay4/1
  Delay3/1 -> Delay2/1, Inner Product/2(v)
  Delay5/1 -> Vector / Scalar Divide/2(y)
  Inner Product/2(validOut) -> Delay/1
  validIn/1 -> Delay1/1
  Vector / Scalar Divide/2(validOut) -> validOut/1
  Delay1/1 -> Inner Product/3(validIn)
  Delay2/1 -> Delay6/1

== system MVDR_example_hdl_4x4_partial_systolic/MVDR HDL/Compute Weight Vector/Serialize Input Data/Output Selector ==
  idx : Inport
  first : Inport  Port=2
  dataIn : Inport  Port=3
  Multiport Switch : MultiPortSwitch  DataPortOrder=Zero-based contiguous  Inputs=4  zeroidx=on
  Row 1 : Selector  NumberOfDimensions=2  InputPortWidth=3  IndexOptions=Index vector (dialog),Select all  Indices=1,1  OutputSizes=1,1
  Row 2 : Selector  NumberOfDimensions=2  InputPortWidth=3  IndexOptions=Index vector (dialog),Select all  Indices=2,1  OutputSizes=1,1
  Row 3 : Selector  NumberOfDimensions=2  InputPortWidth=3  IndexOptions=Index vector (dialog),Select all  Indices=3,1  OutputSizes=1,1
  Row 4 : Selector  NumberOfDimensions=2  InputPortWidth=3  IndexOptions=Index vector (dialog),Select all  Indices=4,1  OutputSizes=1,1
  Unit Delay Enabled Synchronous : hdlsllib/Discrete/Unit Delay Enabled Synchronous  InitialCondition=0.0  SampleTime=-1
      settings: SourceProductBaseCode=SL
  dataOut : Outport
  wires:
  Row 1/1 -> Multiport Switch/2
  Row 4/1 -> Multiport Switch/5
  Unit Delay Enabled Synchronous/1 -> Row 4/1, Row 3/1, Row 2/1
  dataIn/1 -> Unit Delay Enabled Synchronous/1, Row 1/1
  Row 2/1 -> Multiport Switch/3
  idx/1 -> Multiport Switch/1
  Row 3/1 -> Multiport Switch/4
  Multiport Switch/1 -> dataOut/1
  first/1 -> Unit Delay Enabled Synchronous/2

== system MVDR_example_hdl_4x4_partial_systolic/MVDR HDL/Compute Weight Vector/Serialize Input Data/Output Selector1 ==
  idx : Inport
  first : Inport  Port=2
  dataIn : Inport  Port=3
  Multiport Switch : MultiPortSwitch  DataPortOrder=Zero-based contiguous  Inputs=4  zeroidx=on
  Row 1 : Selector  NumberOfDimensions=2  InputPortWidth=3  IndexOptions=Index vector (dialog),Select all  Indices=1,1  OutputSizes=1,1
  Row 2 : Selector  NumberOfDimensions=2  InputPortWidth=3  IndexOptions=Index vector (dialog),Select all  Indices=2,1  OutputSizes=1,1
  Row 3 : Selector  NumberOfDimensions=2  InputPortWidth=3  IndexOptions=Index vector (dialog),Select all  Indices=3,1  OutputSizes=1,1
  Row 4 : Selector  NumberOfDimensions=2  InputPortWidth=3  IndexOptions=Index vector (dialog),Select all  Indices=4,1  OutputSizes=1,1
  Unit Delay Enabled Synchronous : hdlsllib/Discrete/Unit Delay Enabled Synchronous  InitialCondition=0.0  SampleTime=-1
      settings: SourceProductBaseCode=SL
  dataOut : Outport
  wires:
  first/1 -> Unit Delay Enabled Synchronous/2
  Multiport Switch/1 -> dataOut/1
  Row 3/1 -> Multiport Switch/4
  idx/1 -> Multiport Switch/1
  Row 2/1 -> Multiport Switch/3
  dataIn/1 -> Row 1/1, Unit Delay Enabled Synchronous/1
  Unit Delay Enabled Synchronous/1 -> Row 2/1, Row 3/1, Row 4/1
  Row 4/1 -> Multiport Switch/5
  Row 1/1 -> Multiport Switch/2

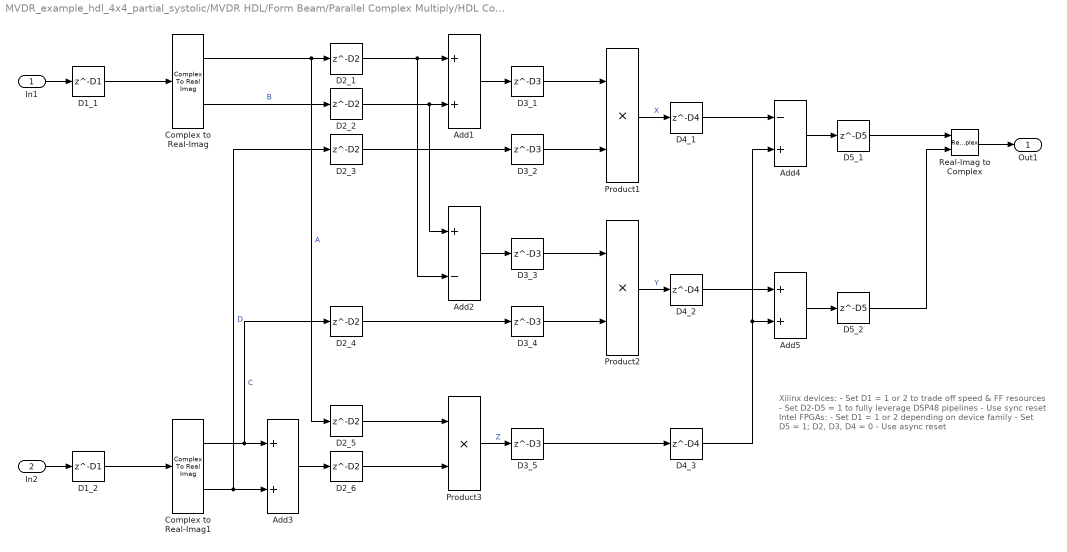
== system MVDR_example_hdl_4x4_partial_systolic/MVDR HDL/Form Beam/Parallel Complex Multiply/HDL Complex Multiply ==
  note: Xilinx devices:
      | - Set D1 = 1 or 2 to trade off speed & FF resources
      | - Set D2-D5 = 1 to fully leverage DSP48 pipelines
      | - Use sync reset
      |
      | Intel FPGAs:
      | - Set D1 = 1 or 2 depending on device family
      | - Set D5 = 1; D2, D3, D4 = 0
      | - Use async reset
  In1 : Inport
  In2 : Inport  Port=2
  Add1 : Sum
  Add2 : Sum  Inputs=+-
  Add3 : Sum
  Add4 : Sum  Inputs=-+
  Add5 : Sum
  Complex to Real-Imag : ComplexToRealImag
  Complex to Real-Imag1 : ComplexToRealImag
  D1_1 : Delay  DelayLength=D1
  D1_2 : Delay  DelayLength=D1
  D2_{1..6} (6 alike) : Delay  DelayLength=D2
  D3_{1..5} (5 alike) : Delay  DelayLength=D3
  D4_1 : Delay  DelayLength=D4
  D4_2 : Delay  DelayLength=D4
  D4_3 : Delay  DelayLength=D4
  D5_1 : Delay  DelayLength=D5
  D5_2 : Delay  DelayLength=D5
  Product1 : Product
  Product2 : Product
  Product3 : Product
  Real-Imag to Complex : RealImagToComplex
  Out1 : Outport  VectorParamsAs1DForOutWhenUnconnected=off
  wires:
  Real-Imag to Complex/1 -> Out1/1
  In2/1 -> D1_2/1
  Complex to Real-Imag1/1 -> Add3/1, D2_4/1  "C"
  Complex to Real-Imag1/2 -> Add3/2, D2_3/1  "D"
  Product1/1 -> D4_1/1  "X"
  Product2/1 -> D4_2/1  "Y"
  Product3/1 -> D3_5/1  "Z"
  Add4/1 -> D5_1/1
  Add5/1 -> D5_2/1
  D5_1/1 -> Real-Imag to Complex/1
  D5_2/1 -> Real-Imag to Complex/2
  D4_1/1 -> Add4/1
  D4_2/1 -> Add5/1
  D3_5/1 -> D4_3/1
  Add1/1 -> D3_1/1
  Add3/1 -> D2_6/1
  Add2/1 -> D3_3/1
  Complex to Real-Imag/1 -> D2_5/1, D2_1/1  "A"
  Complex to Real-Imag/2 -> D2_2/1  "B"
  D3_1/1 -> Product1/1
  D2_6/1 -> Product3/2
  D3_3/1 -> Product2/1
  D4_3/1 -> Add4/2, Add5/2
  D3_4/1 -> Product2/2
  D3_2/1 -> Product1/2
  D2_4/1 -> D3_4/1
  D2_3/1 -> D3_2/1
  D2_5/1 -> Product3/1
  D2_2/1 -> Add1/2, Add2/1
  D2_1/1 -> Add2/2, Add1/1
  In1/1 -> D1_1/1
  D1_1/1 -> Complex to Real-Imag/1
  D1_2/1 -> Complex to Real-Imag1/1

== system MVDR_example_hdl_4x4_partial_systolic/MVDR HDL/Form Covariance Matrix/Matrix Multiply Partitioned/Partition x_conj ==
  x : Inport
  x_conj : Inport  Port=2  Partition=on  PartitionDimension=1  PartitionWidth=1  PartitionOffset=0
  For Each : ForEach  DisableCoverage=on
  Partition x : Subsystem  TreatAsAtomicUnit=on
  C : Outport  ConcatenationDimension=1
  wires:
  x_conj/1 -> Partition x/2(x_conj_elem)
  x/1 -> Partition x/1(x)
  Partition x/1(C_col) -> C/1

== system MVDR_example_hdl_4x4_partial_systolic/MVDR HDL/Normalize Response/MVDR Weight Update/Inner Product ==
  u : Inport
  v : Inport  Port=2
  validIn : Inport  Port=3
  Conjugate : Math  Operator=conj  SignedPower=on  RndMeth=Zero  SaturateOnIntegerOverflow=on
  Delay : Delay  DelayLength=1
  Delay1 : Delay  DelayLength=6
  Delay2 : Delay  DelayLength=ceil(log2(numArrayElements))
  Delay4 : Delay  DelayLength=1
  Element-wise complex product : Subsystem  TreatAsAtomicUnit=on
  Tree Sum with Distributed Pipelining : Subsystem
  y : Outport
  validOut : Outport  Port=2
  wires:
  v/1 -> Conjugate/1
  u/1 -> Element-wise complex product/2(v)
  validIn/1 -> Delay1/1
  Element-wise complex product/1(y) -> Delay/1
  Delay2/1 -> validOut/1
  Delay1/1 -> Delay4/1
  Delay4/1 -> Delay2/1
  Conjugate/1 -> Element-wise complex product/1(u)
  Delay/1 -> Tree Sum with Distributed Pipelining/1(In1)
  Tree Sum with Distributed Pipelining/1(Out1) -> y/1

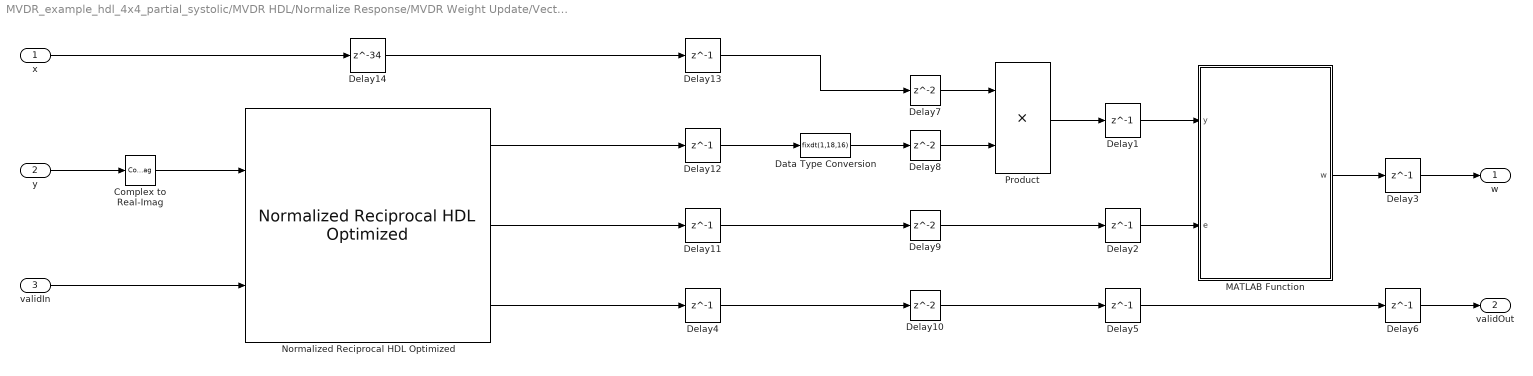
== system MVDR_example_hdl_4x4_partial_systolic/MVDR HDL/Normalize Response/MVDR Weight Update/Vector // Scalar Divide ==
  x : Inport
  y : Inport  Port=2
  validIn : Inport  Port=3
  Complex to Real-Imag : ComplexToRealImag  Output=Real
  Data Type Conversion : DataTypeConversion  OutDataTypeStr=fixdt(1,18,16)
  Delay{1..6,11..13} (9 alike) : Delay  DelayLength=1
  Delay{7..10} (4 alike) : Delay
  Delay14 : Delay  DelayLength=34
  MATLAB Function : MATLAB Function  TreatAsAtomicUnit=on
  Normalized Reciprocal HDL Optimized : embreciprocals/Normalized Reciprocal HDL Optimized
      settings: SourceProductBaseCode=SL
  Product : Product  OutDataTypeStr=Inherit: Same as first input
  w : Outport
  validOut : Outport  Port=2
  wires:
  Delay2/1 -> MATLAB Function/2(e)
  y/1 -> Complex to Real-Imag/1
  Delay12/1 -> Data Type Conversion/1
  Complex to Real-Imag/1 -> Normalized Reciprocal HDL Optimized/1
  Delay13/1 -> Delay7/1
  Normalized Reciprocal HDL Optimized/2 -> Delay11/1
  Normalized Reciprocal HDL Optimized/1 -> Delay12/1
  Delay1/1 -> MATLAB Function/1(y)
  validIn/1 -> Normalized Reciprocal HDL Optimized/2
  Product/1 -> Delay1/1
  Delay11/1 -> Delay9/1
  MATLAB Function/1(w) -> Delay3/1
  Normalized Reciprocal HDL Optimized/3 -> Delay4/1
  Delay3/1 -> w/1
  Delay4/1 -> Delay10/1
  Delay5/1 -> Delay6/1
  Delay6/1 -> validOut/1
  x/1 -> Delay14/1
  Data Type Conversion/1 -> Delay8/1
  Delay7/1 -> Product/1
  Delay8/1 -> Product/2
  Delay9/1 -> Delay2/1
  Delay10/1 -> Delay5/1
  Delay14/1 -> Delay13/1

== system MVDR_example_hdl_4x4_partial_systolic/MVDR HDL/Form Covariance Matrix/Matrix Multiply Partitioned/Partition x_conj/Partition x ==
  x : Inport  Partition=on  PartitionDimension=1  PartitionWidth=1  PartitionOffset=0
  x_conj_elem : Inport  Port=2
  For Each : ForEach  DisableCoverage=on
  HDL Complex Multiply : Subsystem  mask(HDL Complex Multiplier (3 Multiply, 5 Add)){D1=2, D2=1, D3=1, D4=1, D5=1}
      mask help:
      | Xilinx devices:
      | - Set D1 = 1 or 2 to trade off speed & FF resources
      | - Set D2-D5 = 1 to fully leverage DSP48 pipelines
      | - Use sync reset
      |
      | Intel FPGAs:
      | - Set D1 = 1 or 2 depending on device family
      | - Set D5 = 1; D2, D3, D4 = 0
      | - Use async reset
      mask init:
      | delay = D1+D2+D3+D4+D5;
      mask Display:
      | fprintf('Delay=%d',delay);
      | port_label('input',1,'z1');
      | port_label('input',2,'z2');
  C_col : Outport  ConcatenationDimension=1
  wires:
  x/1 -> HDL Complex Multiply/1(In1)
  x_conj_elem/1 -> HDL Complex Multiply/2(In2)
  HDL Complex Multiply/1(Out1) -> C_col/1

== system MVDR_example_hdl_4x4_partial_systolic/MVDR HDL/Normalize Response/MVDR Weight Update/Inner Product/Element-wise complex product ==
  u : Inport  Partition=on  PartitionDimension=1  PartitionWidth=1  PartitionOffset=0
  v : Inport  Port=2  Partition=on  PartitionDimension=1  PartitionWidth=1  PartitionOffset=0
  For Each : ForEach  DisableCoverage=on
  HDL Complex Multiply : Subsystem  mask(HDL Complex Multiplier (3 Multiply, 5 Add)){D1=2, D2=1, D3=1, D4=1, D5=1}
      mask help:
      | Xilinx devices:
      | - Set D1 = 1 or 2 to trade off speed & FF resources
      | - Set D2-D5 = 1 to fully leverage DSP48 pipelines
      | - Use sync reset
      |
      | Intel FPGAs:
      | - Set D1 = 1 or 2 depending on device family
      | - Set D5 = 1; D2, D3, D4 = 0
      | - Use async reset
      mask init:
      | delay = D1+D2+D3+D4+D5;
      mask Display:
      | fprintf('Delay=%d',delay);
      | port_label('input',1,'z1');
      | port_label('input',2,'z2');
  y : Outport  ConcatenationDimension=1
  wires:
  v/1 -> HDL Complex Multiply/2(In2)
  HDL Complex Multiply/1(Out1) -> y/1
  u/1 -> HDL Complex Multiply/1(In1)

== system MVDR_example_hdl_4x4_partial_systolic/MVDR HDL/Normalize Response/MVDR Weight Update/Inner Product/Tree Sum with Distributed Pipelining ==
  In1 : Inport
  Delay3 : Delay  DelayLength=ceil(log2(numArrayElements))
  Tree Sum of Elements : Sum  Inputs=+  OutDataTypeStr=Inherit: Same as first input  LockScale=on
  Out1 : Outport
  wires:
  Delay3/1 -> Out1/1
  In1/1 -> Tree Sum of Elements/1
  Tree Sum of Elements/1 -> Delay3/1

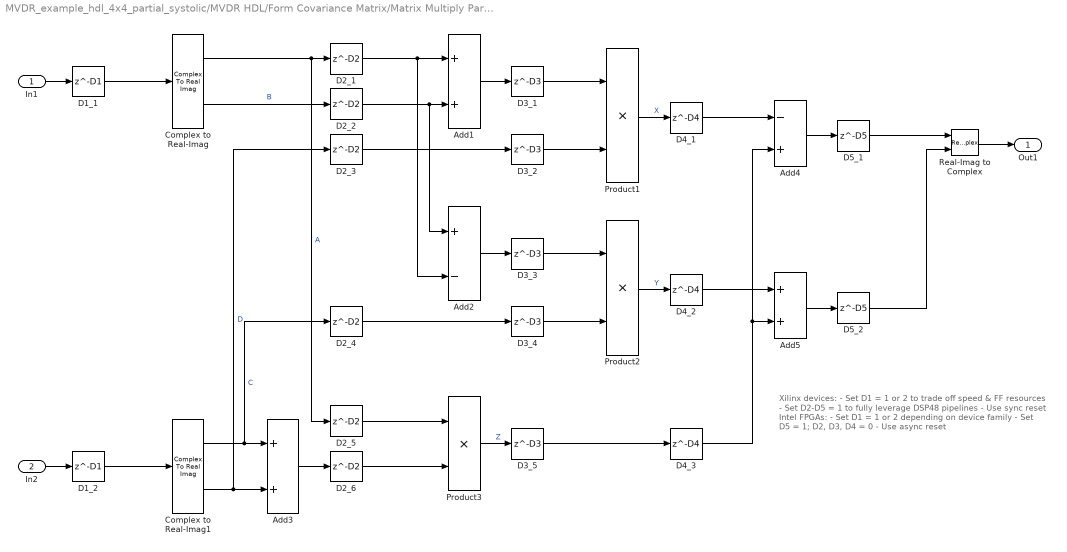
== system MVDR_example_hdl_4x4_partial_systolic/MVDR HDL/Form Covariance Matrix/Matrix Multiply Partitioned/Partition x_conj/Partition x/HDL Complex Multiply ==
  note: Xilinx devices:
      | - Set D1 = 1 or 2 to trade off speed & FF resources
      | - Set D2-D5 = 1 to fully leverage DSP48 pipelines
      | - Use sync reset
      |
      | Intel FPGAs:
      | - Set D1 = 1 or 2 depending on device family
      | - Set D5 = 1; D2, D3, D4 = 0
      | - Use async reset
  In1 : Inport
  In2 : Inport  Port=2
  Add1 : Sum
  Add2 : Sum  Inputs=+-
  Add3 : Sum
  Add4 : Sum  Inputs=-+
  Add5 : Sum
  Complex to Real-Imag : ComplexToRealImag
  Complex to Real-Imag1 : ComplexToRealImag
  D1_1 : Delay  DelayLength=D1
  D1_2 : Delay  DelayLength=D1
  D2_{1..6} (6 alike) : Delay  DelayLength=D2
  D3_{1..5} (5 alike) : Delay  DelayLength=D3
  D4_1 : Delay  DelayLength=D4
  D4_2 : Delay  DelayLength=D4
  D4_3 : Delay  DelayLength=D4
  D5_1 : Delay  DelayLength=D5
  D5_2 : Delay  DelayLength=D5
  Product1 : Product
  Product2 : Product
  Product3 : Product
  Real-Imag to Complex : RealImagToComplex
  Out1 : Outport  VectorParamsAs1DForOutWhenUnconnected=off
  wires:
  Real-Imag to Complex/1 -> Out1/1
  In2/1 -> D1_2/1
  Complex to Real-Imag1/1 -> Add3/1, D2_4/1  "C"
  Complex to Real-Imag1/2 -> Add3/2, D2_3/1  "D"
  Product1/1 -> D4_1/1  "X"
  Product2/1 -> D4_2/1  "Y"
  Product3/1 -> D3_5/1  "Z"
  Add4/1 -> D5_1/1
  Add5/1 -> D5_2/1
  D5_1/1 -> Real-Imag to Complex/1
  D5_2/1 -> Real-Imag to Complex/2
  D4_1/1 -> Add4/1
  D4_2/1 -> Add5/1
  D3_5/1 -> D4_3/1
  Add1/1 -> D3_1/1
  Add3/1 -> D2_6/1
  Add2/1 -> D3_3/1
  Complex to Real-Imag/1 -> D2_5/1, D2_1/1  "A"
  Complex to Real-Imag/2 -> D2_2/1  "B"
  D3_1/1 -> Product1/1
  D2_6/1 -> Product3/2
  D3_3/1 -> Product2/1
  D4_3/1 -> Add4/2, Add5/2
  D3_4/1 -> Product2/2
  D3_2/1 -> Product1/2
  D2_4/1 -> D3_4/1
  D2_3/1 -> D3_2/1
  D2_5/1 -> Product3/1
  D2_2/1 -> Add1/2, Add2/1
  D2_1/1 -> Add2/2, Add1/1
  In1/1 -> D1_1/1
  D1_1/1 -> Complex to Real-Imag/1
  D1_2/1 -> Complex to Real-Imag1/1

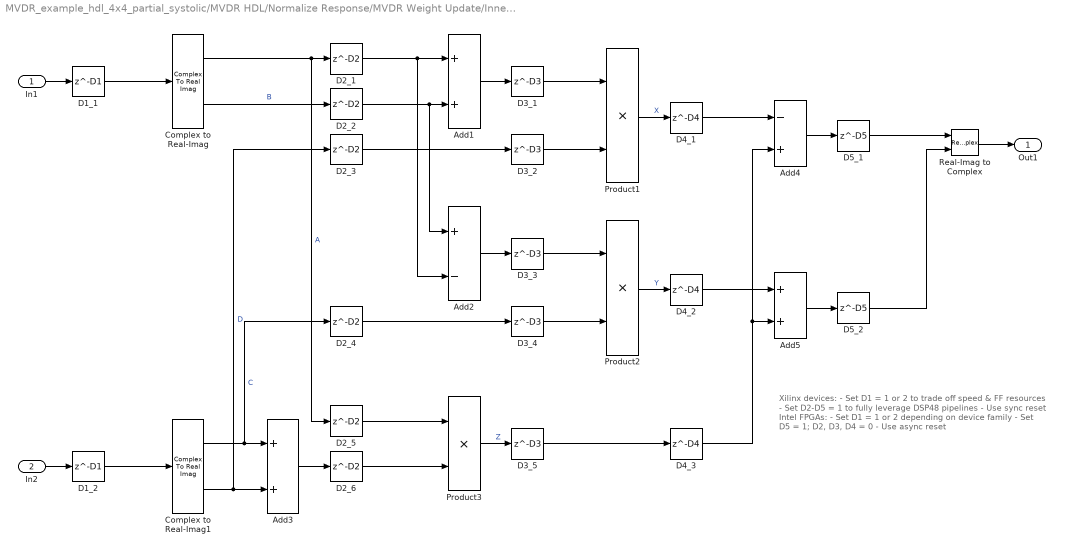
== system MVDR_example_hdl_4x4_partial_systolic/MVDR HDL/Normalize Response/MVDR Weight Update/Inner Product/Element-wise complex product/HDL Complex Multiply ==
  note: Xilinx devices:
      | - Set D1 = 1 or 2 to trade off speed & FF resources
      | - Set D2-D5 = 1 to fully leverage DSP48 pipelines
      | - Use sync reset
      |
      | Intel FPGAs:
      | - Set D1 = 1 or 2 depending on device family
      | - Set D5 = 1; D2, D3, D4 = 0
      | - Use async reset
  In1 : Inport
  In2 : Inport  Port=2
  Add1 : Sum
  Add2 : Sum  Inputs=+-
  Add3 : Sum
  Add4 : Sum  Inputs=-+
  Add5 : Sum
  Complex to Real-Imag : ComplexToRealImag
  Complex to Real-Imag1 : ComplexToRealImag
  D1_1 : Delay  DelayLength=D1
  D1_2 : Delay  DelayLength=D1
  D2_{1..6} (6 alike) : Delay  DelayLength=D2
  D3_{1..5} (5 alike) : Delay  DelayLength=D3
  D4_1 : Delay  DelayLength=D4
  D4_2 : Delay  DelayLength=D4
  D4_3 : Delay  DelayLength=D4
  D5_1 : Delay  DelayLength=D5
  D5_2 : Delay  DelayLength=D5
  Product1 : Product  OutDataTypeStr=Inherit: Same as first input
  Product2 : Product  OutDataTypeStr=Inherit: Same as first input
  Product3 : Product  OutDataTypeStr=Inherit: Same as first input
  Real-Imag to Complex : RealImagToComplex
  Out1 : Outport  VectorParamsAs1DForOutWhenUnconnected=off
  wires:
  Real-Imag to Complex/1 -> Out1/1
  In2/1 -> D1_2/1
  Complex to Real-Imag1/1 -> Add3/1, D2_4/1  "C"
  Complex to Real-Imag1/2 -> Add3/2, D2_3/1  "D"
  Product1/1 -> D4_1/1  "X"
  Product2/1 -> D4_2/1  "Y"
  Product3/1 -> D3_5/1  "Z"
  Add4/1 -> D5_1/1
  Add5/1 -> D5_2/1
  D5_1/1 -> Real-Imag to Complex/1
  D5_2/1 -> Real-Imag to Complex/2
  D4_1/1 -> Add4/1
  D4_2/1 -> Add5/1
  D3_5/1 -> D4_3/1
  Add1/1 -> D3_1/1
  Add3/1 -> D2_6/1
  Add2/1 -> D3_3/1
  Complex to Real-Imag/1 -> D2_5/1, D2_1/1  "A"
  Complex to Real-Imag/2 -> D2_2/1  "B"
  D3_1/1 -> Product1/1
  D2_6/1 -> Product3/2
  D3_3/1 -> Product2/1
  D4_3/1 -> Add4/2, Add5/2
  D3_4/1 -> Product2/2
  D3_2/1 -> Product1/2
  D2_4/1 -> D3_4/1
  D2_3/1 -> D3_2/1
  D2_5/1 -> Product3/1
  D2_2/1 -> Add1/2, Add2/1
  D2_1/1 -> Add2/2, Add1/1
  In1/1 -> D1_1/1
  D1_1/1 -> Complex to Real-Imag/1
  D1_2/1 -> Complex to Real-Imag1/1

== matlab function MVDR_example_hdl_4x4_partial_systolic/MVDR MATLAB/MATLAB Function ==
  data: X input; Y output; sv parameter
function Y = mvdr_beamform(X, sv)

% form covariance matrix
Ecx = X.'*conj(X);

% compute weight vector
wp = Ecx\sv;

% normalize response
w = wp/(sv'*wp);

% form output beam
Y = X*conj(w);

end

== matlab function MVDR_example_hdl_4x4_partial_systolic/MVDR HDL/Compute Weight Vector/Serialize Input Data/readyQueue ==
  data: readyEdge input; validOut output; validIn input
function validOut = readyQueue(readyEdge, validIn)

persistent readyQueued_reg
if isempty(readyQueued_reg)
    readyQueued_reg = false;
end

readyQueued = readyQueued_reg;

if readyEdge
    if validIn
        validOut = true;
    else
        validOut = false;
        readyQueued_reg = true;
    end
elseif readyQueued
    if validIn
        validOut = true;
        readyQueued_reg = false;
    else
        validOut = false; 
    end
else
    validOut = false;
end

== matlab function MVDR_example_hdl_4x4_partial_systolic/MVDR HDL/Normalize Response/MVDR Weight Update/Vector // Scalar Divide/MATLAB Function ==
  data: y input; w output; e input
function w = variableShift(y,e)
    %#codegen
    w = bitshift(y,e);
end

function C = bitshift(A,K)
%BITSHIFT Bit-wise shift.
%   C = bitshift(A, K) returns the value of fi object A
%   shifted by K bits, in fi object C.  fi object A can be any
%   fixed-point numeric type, and may either be a scalar or a
%   vector. K must be a scalar with built-in type. The
%   OverflowAction property is obeyed. The RoundingMethod is always
%   'Floor'.  
%
%   Behavior shifting off the top and bottom: If K > A.WordLength,
%   then C = upperbound(A).  If K is negative and -K >
%   A.WordLength, then C = 0.
%
%   If A is not a fi object, then C = A .* 2.^K.
    coder.inline('never')
    if isfi(A)
        if K>0
            if K>(A.WordLength-1)
                C = zeros(size(A),'like',A);
                C(:) = upperbound(A);
            else
                C = bitsll(A,K);
            end
        else
            if -K>(A.WordLength-1)
                C = zeros(size(A),'like',A);
            else
                C = bitsra(A,-K);
            end
        end
    else
        C = cast(double(A) .* 2.^double(K),'like',A);
    end
end
